simulink model "mobileRobotAPI"  (R2025a)
settings: Solver=VariableStepAuto  StartTime=0.0  StopTime=10.0  RelTol=1e-3
settings Model: DataDictionary=SensorInterfaces.sldd  Creator=Rasika Kale  LastModifiedBy=Rasika Kale

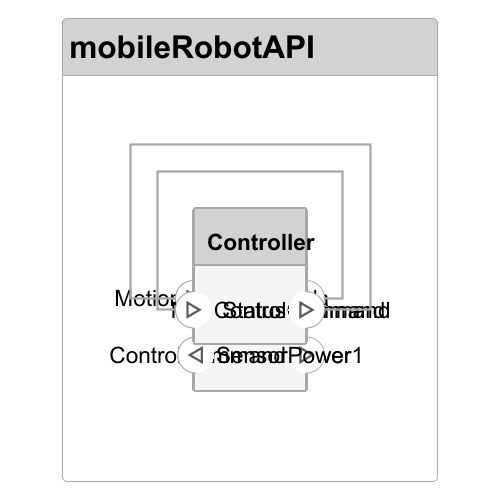
[thumbnail: Simulink's stored preview of the top-level diagram]
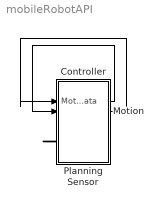
== system mobileRobotAPI ==
  Controller : Subsystem
      settings: PortSchema="{\"entries\":[{\"content\":{\"headerSize\":26,\"margin\":15,\"minimumSpacing\":25,\"sides\":[{\"content\":{\"connectorIds\":[\"In1\"]},\"type\":\"ConnectorPlacement.EquallySpacedRectSide\",\"uuid\":\"ddc0c878-bcd3-4a9e-acff-828786b6ea84\"},{\"content\":{\"connectorIds\":[\"Out1\"],\"side\":\"RIGHT\"},\"type\":\"ConnectorPlacement.EquallySpacedRectSide\",\"uuid\":\"828fb2d0-888b-4c08-9d3f-4ba7b8b66689\"},{\"content\":{\"side\":\"TOP\"},\"type\":\"ConnectorPlacement.EquallySpacedRectSide\",\"uuid\":\"e50699e1-3d97-445e-97d1-81cfb175c7da\"}]},\"type\":\"ConnectorPlacement.EquallySpacedConnector\",\"uuid\":\"272472d2-7a17-4bee-a371-679485dcccc3\"}],\"packageUris\":[\"http://schema.mathworks.com/mf0/Connector/R2020b\"],\"version\":\"1.0\"}"
  Motion : Subsystem
      settings: PortSchema="{\"entries\":[{\"content\":{\"headerSize\":26,\"margin\":15,\"minimumSpacing\":25,\"sides\":[{\"content\":{\"connectorIds\":[\"In1\"]},\"type\":\"ConnectorPlacement.EquallySpacedRectSide\",\"uuid\":\"ddc0c878-bcd3-4a9e-acff-828786b6ea84\"},{\"content\":{\"connectorIds\":[\"Out1\"],\"side\":\"RIGHT\"},\"type\":\"ConnectorPlacement.EquallySpacedRectSide\",\"uuid\":\"828fb2d0-888b-4c08-9d3f-4ba7b8b66689\"},{\"content\":{\"side\":\"TOP\"},\"type\":\"ConnectorPlacement.EquallySpacedRectSide\",\"uuid\":\"e50699e1-3d97-445e-97d1-81cfb175c7da\"}]},\"type\":\"ConnectorPlacement.EquallySpacedConnector\",\"uuid\":\"272472d2-7a17-4bee-a371-679485dcccc3\"}],\"packageUris\":[\"http://schema.mathworks.com/mf0/Connector/R2020b\"],\"version\":\"1.0\"}"
  Planning : Subsystem
      settings: PortSchema="{\"entries\":[{\"content\":{\"headerSize\":26,\"margin\":15,\"minimumSpacing\":25,\"sides\":[{\"content\":{\"connectorIds\":[\"In1\",\"LConn1\"]},\"type\":\"ConnectorPlacement.EquallySpacedRectSide\",\"uuid\":\"ddc0c878-bcd3-4a9e-acff-828786b6ea84\"},{\"content\":{\"connectorIds\":[\"Out1\",\"Out2\"],\"side\":\"RIGHT\"},\"type\":\"ConnectorPlacement.EquallySpacedRectSide\",\"uuid\":\"828fb2d0-888b-4c08-9d3f-4ba7b8b66689\"},{\"content\":{\"side\":\"TOP\"},\"type\":\"ConnectorPlacement.EquallySpacedRectSide\",\"uuid\":\"e50699e1-3d97-445e-97d1-81cfb175c7da\"}]},\"type\":\"ConnectorPlacement.EquallySpacedConnector\",\"uuid\":\"272472d2-7a17-4bee-a371-679485dcccc3\"}],\"packageUris\":[\"http://schema.mathworks.com/mf0/Connector/R2020b\"],\"version\":\"1.0\"}"
  Sensor : Subsystem
      settings: PortSchema="{\"entries\":[{\"content\":{\"headerSize\":26,\"margin\":15,\"minimumSpacing\":25,\"sides\":[{\"content\":{\"connectorIds\":[\"In1\",\"LConn1\"]},\"type\":\"ConnectorPlacement.EquallySpacedRectSide\",\"uuid\":\"ddc0c878-bcd3-4a9e-acff-828786b6ea84\"},{\"content\":{\"side\":\"RIGHT\"},\"type\":\"ConnectorPlacement.EquallySpacedRectSide\",\"uuid\":\"828fb2d0-888b-4c08-9d3f-4ba7b8b66689\"},{\"content\":{\"side\":\"TOP\"},\"type\":\"ConnectorPlacement.EquallySpacedRectSide\",\"uuid\":\"e50699e1-3d97-445e-97d1-81cfb175c7da\"}]},\"type\":\"ConnectorPlacement.EquallySpacedConnector\",\"uuid\":\"272472d2-7a17-4bee-a371-679485dcccc3\"}],\"packageUris\":[\"http://schema.mathworks.com/mf0/Connector/R2020b\"],\"version\":\"1.0\"}"
  wires:
  Motion/1(MotionData) -> Sensor/1(MotionData)
  Planning/1(MotionCommand) -> Motion/1(MotionCommand)
  connections:
  Sensor/LConn1 -- Planning/LConn1

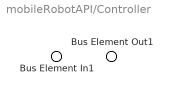
== system mobileRobotAPI/Controller ==
  Bus Element In1 : Inport  PortName=ControlCommand
  Bus Element Out1 : Outport  PortName=Status

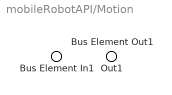
== system mobileRobotAPI/Motion ==
  Bus Element In1 : Inport  PortName=MotionCommand
  Bus Element Out1 : Outport  PortName=MotionData  Element=elem0
  Out1 : Outport  PortName=MotionData  Element=Rotation

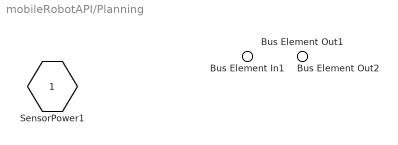
== system mobileRobotAPI/Planning ==
  Bus Element In1 : Inport  PortName=Command
  SensorPower1 : PMIOPort  Side=Left  ConnectionType=Bus: PhysicalInterface
  Bus Element Out1 : Outport  PortName=MotionCommand
  Bus Element Out2 : Outport  Port=2  PortName=ControlCommand

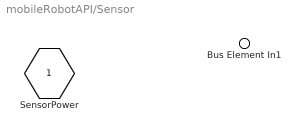
== system mobileRobotAPI/Sensor ==
  Bus Element In1 : Inport  PortName=MotionData
  SensorPower : PMIOPort  Side=Left  ConnectionType=Bus: PhysicalInterface
